simulink model "DYNctl_ver4_etud_obfusc"  (R2015a)
settings: Solver=ode45  StartTime=0.0  StopTime=tfin  FixedStep=0.001  RelTol=1e-09
values from neighbouring files (symbols this model uses):
  A_phi = [A13_13([1 4 11],1),A13_13([1 4 11],4),A13_13([1 4 11],11)]    [SM_4.m]
  A_theta = [A13_13([2 5 12],2),A13_13([2 5 12],5),A13_13([2 5 12],12)]    [SM_4.m]
  A_z = [A13_13([3 6 13],3),A13_13([3 6 13],6),A13_13([3 6 13],13)]    [SM_4.m]
  AxS = [A13_13([7 9],7),A13_13([7 9],9)]    [SM_4.m]
  AyS = [A13_13([8 10],8),A13_13([8 10],10)]    [SM_4.m]
  B_phi = [B13_3([1 4 11],1)]    [SM_4.m]
  B_theta = [B13_3([2 5 12],2)]    [SM_4.m]
  B_z = [B13_3([3 6 13],3)]    [SM_4.m]
  BxS = [0; acc]    [SM_4.m]
  ByS = [-acc; 0]    [SM_4.m]
  C3_3_iden = eye(3)    [SM_4.m]
  CxS = eye(2)    [SM_4.m]
  CyS = eye(2)    [SM_4.m]
  D_phi = [0;0;0]    [SM_4.m]
  D_theta = [0;0;0]    [SM_4.m]
  D_z = [0;0;0]    [SM_4.m]
  DxS = [0;0]    [SM_4.m]
  DyS = [0;0]    [SM_4.m]
  U_inv = 1/(YA*(-XB+XC)+YB*(XA-XC)+YC*(-XA+XB))*[-XB+XC, YC-YB, -YB*XC+YC*XB ... (first row only)    [SM_4.m]
  XA = r_ABC    (= 0.0952)    [SM-4.m]
  XB = -r_ABC*sind(30)    [SM-4.m]
  XC = 0    [SM-4.m]
  YA = 0    [SM-4.m]
  YB = r_ABC*cosd(30)    [SM-4.m]
  YC = -r_ABC*cosd(30)    [SM-4.m]
undefined symbols (not defined in the file or in its folder): ia_e, ib_e, ic_e, phi_e, TABC_trans, TDEF_trans, theta_e, va_e, vb_e, vc_e, vx_s_e, vy_s_e, vz_e, w_phi_e, w_theta_e, x_s_e, y_s_e, z_e
settings Model: CovSFcnEnable=off  Creator=delafontaine  LastModifiedBy=Julien
settings SolverCC: AlgebraicLoopSolver=LineSearch
settings DataIOCC: SignalLoggingSaveFormat=ModelDataLogs
settings DebuggingCC: UnderspecifiedInitializationDetection=Classic  MergeDetectMultiDrivingBlocksExec=none  MultiTaskDSMMsg=warning  MultiTaskCondExecSysMsg=none

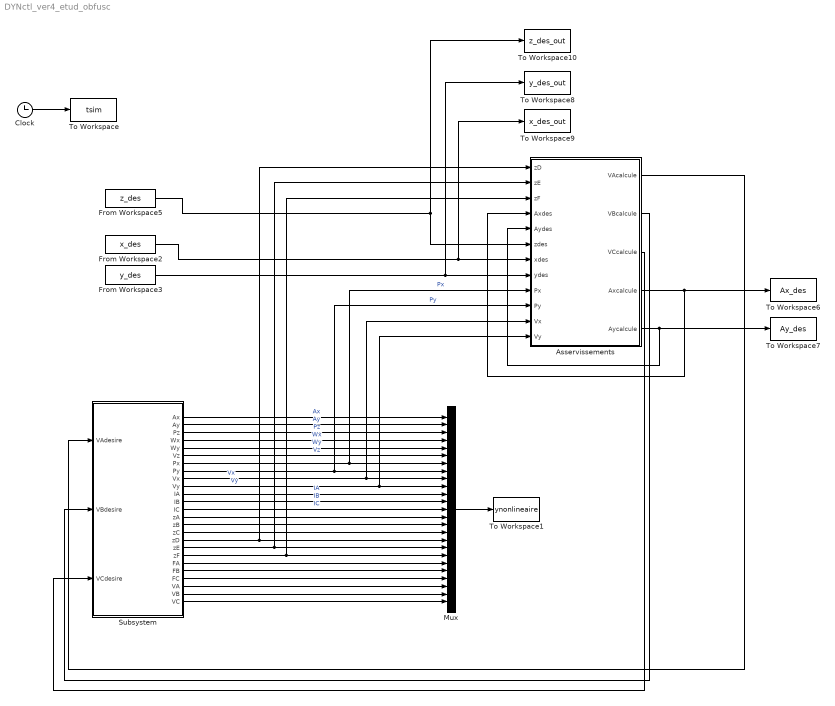
== system DYNctl_ver4_etud_obfusc ==
  Asservissements : Subsystem
      mask help: Simulink:masks:GenSFuncDesc_MD
      mask Help: eval('feval(''rtwprivate'',''rtwhelpview'',''rtw_sfcn_block'')');
  Clock : Clock
  From Workspace2 : FromWorkspace  VariableName=x_des  SampleTime=0  Interpolate=off  OutputAfterFinalValue=Holding final value
  From Workspace3 : FromWorkspace  VariableName=y_des  SampleTime=0  Interpolate=off  OutputAfterFinalValue=Holding final value
  From Workspace5 : FromWorkspace  VariableName=z_des  SampleTime=0  Interpolate=off  OutputAfterFinalValue=Holding final value
  Mux : Mux  Inputs=25
  Subsystem : Subsystem
  To Workspace : ToWorkspace  VariableName=tsim  SampleTime=-1
  To Workspace1 : ToWorkspace  VariableName=ynonlineaire  SampleTime=-1
  To Workspace10 : ToWorkspace  VariableName=z_des_out  SampleTime=-1
  To Workspace6 : ToWorkspace  VariableName=Ax_des  SampleTime=-1
  To Workspace7 : ToWorkspace  VariableName=Ay_des  SampleTime=-1
  To Workspace8 : ToWorkspace  VariableName=y_des_out  SampleTime=-1
  To Workspace9 : ToWorkspace  VariableName=x_des_out  SampleTime=-1
  wires:
  Mux/1 -> To Workspace1/1
  Clock/1 -> To Workspace/1
  From Workspace5/1 -> Asservissements/6(zdes), To Workspace10/1
  Subsystem/1(Ax) -> Mux/1  "Ax"
  Subsystem/2(Ay) -> Mux/2  "Ay"
  Subsystem/3(Pz) -> Mux/3  "Pz"
  Subsystem/4(Wx) -> Mux/4  "Wx"
  Subsystem/5(Wy) -> Mux/5  "Wy"
  Subsystem/6(Vz) -> Mux/6  "Vz"
  Subsystem/7(Px) -> Asservissements/9(Px), Mux/7  "Px"
  Subsystem/8(Py) -> Asservissements/10(Py), Mux/8  "Py"
  Subsystem/9(Vx) -> Asservissements/11(Vx), Mux/9  "Vx"
  Subsystem/10(Vy) -> Asservissements/12(Vy), Mux/10  "Vy"
  Subsystem/11(IA) -> Mux/11  "IA"
  Subsystem/12(IB) -> Mux/12  "IB"
  Subsystem/13(IC) -> Mux/13  "IC"
  From Workspace3/1 -> Asservissements/8(ydes), To Workspace8/1
  From Workspace2/1 -> Asservissements/7(xdes), To Workspace9/1
  Subsystem/20(FA) -> Mux/20
  Subsystem/21(FB) -> Mux/21
  Subsystem/22(FC) -> Mux/22
  Subsystem/23(VA) -> Mux/23
  Subsystem/24(VB) -> Mux/24
  Subsystem/25(VC) -> Mux/25
  Subsystem/17(zD) -> Asservissements/1(zD), Mux/17
  Subsystem/18(zE) -> Asservissements/2(zE), Mux/18
  Subsystem/19(zF) -> Asservissements/3(zF), Mux/19
  Subsystem/14(zA) -> Mux/14
  Subsystem/15(zB) -> Mux/15
  Subsystem/16(zC) -> Mux/16
  Asservissements/4(Axcalcule) -> Asservissements/4(Axdes), To Workspace6/1
  Asservissements/5(Aycalcule) -> Asservissements/5(Aydes), To Workspace7/1
  Asservissements/1(VAcalcule) -> Subsystem/1(VAdesire)
  Asservissements/2(VBcalcule) -> Subsystem/2(VBdesire)
  Asservissements/3(VCcalcule) -> Subsystem/3(VCdesire)

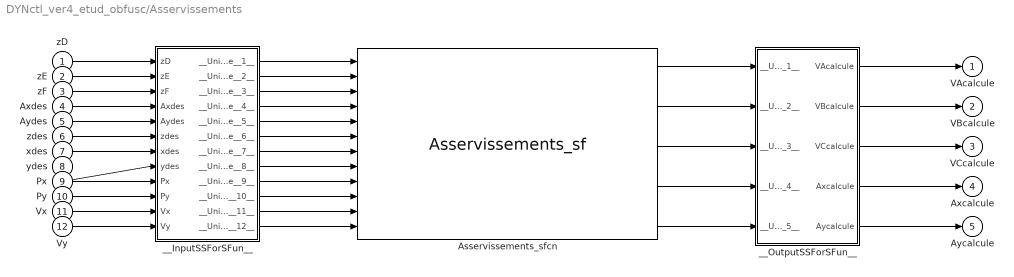
== system DYNctl_ver4_etud_obfusc/Asservissements ==
  zD : Inport
  zE : Inport  Port=2
  zF : Inport  Port=3
  Axdes : Inport  Port=4
  Aydes : Inport  Port=5
  zdes : Inport  Port=6
  xdes : Inport  Port=7
  ydes : Inport  Port=8
  Px : Inport  Port=9
  Py : Inport  Port=10
  Vx : Inport  Port=11
  Vy : Inport  Port=12
  Asservissements_sfcn : S-Function  FunctionName=Asservissements_sf  SFunctionModules=""  mask{rtw_sf_name=Asservissements_sf, showVar=off}
      mask prompts: rtw_sf_name "Simulink:masks:GenSFuncName_MP"; showVar "Simulink:masks:GenSFuncShowModuleList_MP"
      mask help: Simulink:masks:GenSFuncDesc_MD
      mask init:
      | displist = '';
      | if ~strcmp(get_param(gcb, 'FunctionName'), rtw_sf_name);
      |   set_param(gcb, 'FunctionName', rtw_sf_name);
      | end
      | % Check if we are generating code
      | rtw_mode = false;
      | if strcmpi(get_param(bdroot(gcb),'SimulationStatus'),'Initializing')
      | 	rtw_mode = strcmpi(get_param(bdroot(gcb),'BuildingRTWCode'),'on') && ...
      | 		~strcmpi(get_param(bdroot(gcb),'TargetStyle'),'SimulationTarget');
      | end
      | if showVar || rtw_mode
      | 	if exist('rtwsfunc') == 2 | exist('rtwsfunc') == 6
      | 		tmplist = rtwsfunc(rtw_sf_name,gcb);
      | 		tmplist = DAStudio.message('Simulink:masks:GenSFuncListOfModules_IC', tmplist);
      | 	elseif showVar
      | 		tmplist1 = DAStudio.message('Simulink:masks:GenSFuncListOfModules_IC', '');
      |         tmplist2 = DAStudio.message('Simulink:masks:GenSFuncNotLicensed_IC');
      |         tmplist = [tmplist1 tmplist2];
      |  	end
      | end
      | if showVar
      |   displist = tmplist;
      | end
      settings: CopyFcn=|
      | if ~strcmp(get_param(gcb,'Linkstatus'),'none') && ...
      | ~strcmp(get_param(gcb,'Linkstatus'),'implicit')
      |   set_param(gcb,'LinkStatus','none');
      | end
      mask Help: eval('feval(''rtwprivate'',''rtwhelpview'',''rtw_sfcn_block'')');
      mask Display:
      | port_label('input',1,'zD');
      | port_label('input',2,'zE');
      | port_label('input',3,'zF');
      | port_label('input',4,'Axdes');
      | port_label('input',5,'Aydes');
      | port_label('input',6,'zdes');
      | port_label('input',7,'xdes');
      | port_label('input',8,'ydes');
      | port_label('input',9,'Px');
      | port_label('input',10,'Py');
      | port_label('input',11,'Vx');
      | port_label('input',12,'Vy');
      | port_label('output',1,'VAcalcule');
      | port_label('output',2,'VBcalcule');
      | port_label('output',3,'VCcalcule');
      | port_label('output',4,'Axcalcule');
      | port_label('output',5,'Aycalcule');
  __InputSSForSFun__ : Subsystem
  __OutputSSForSFun__ : Subsystem
  VAcalcule : Outport
  VBcalcule : Outport  Port=2
  VCcalcule : Outport  Port=3
  Axcalcule : Outport  Port=4
  Aycalcule : Outport  Port=5
  wires:
  zD/1 -> __InputSSForSFun__/1(zD)
  zE/1 -> __InputSSForSFun__/2(zE)
  zF/1 -> __InputSSForSFun__/3(zF)
  Axdes/1 -> __InputSSForSFun__/4(Axdes)
  Aydes/1 -> __InputSSForSFun__/5(Aydes)
  zdes/1 -> __InputSSForSFun__/6(zdes)
  xdes/1 -> __InputSSForSFun__/7(xdes)
  ydes/1 -> __InputSSForSFun__/8(ydes)
  Px/1 -> __InputSSForSFun__/9(Px)
  Py/1 -> __InputSSForSFun__/10(Py)
  Vx/1 -> __InputSSForSFun__/11(Vx)
  Vy/1 -> __InputSSForSFun__/12(Vy)
  __InputSSForSFun__/1(__UniqueOutportName__1__) -> Asservissements_sfcn/1
  __InputSSForSFun__/2(__UniqueOutportName__2__) -> Asservissements_sfcn/2
  __InputSSForSFun__/3(__UniqueOutportName__3__) -> Asservissements_sfcn/3
  __InputSSForSFun__/4(__UniqueOutportName__4__) -> Asservissements_sfcn/4
  __InputSSForSFun__/5(__UniqueOutportName__5__) -> Asservissements_sfcn/5
  __InputSSForSFun__/6(__UniqueOutportName__6__) -> Asservissements_sfcn/6
  __InputSSForSFun__/7(__UniqueOutportName__7__) -> Asservissements_sfcn/7
  __InputSSForSFun__/8(__UniqueOutportName__8__) -> Asservissements_sfcn/8
  __InputSSForSFun__/9(__UniqueOutportName__9__) -> Asservissements_sfcn/9
  __InputSSForSFun__/10(__UniqueOutportName__10__) -> Asservissements_sfcn/10
  __InputSSForSFun__/11(__UniqueOutportName__11__) -> Asservissements_sfcn/11
  __InputSSForSFun__/12(__UniqueOutportName__12__) -> Asservissements_sfcn/12
  Asservissements_sfcn/1 -> __OutputSSForSFun__/1(__UniqueInportName__1__)
  Asservissements_sfcn/2 -> __OutputSSForSFun__/2(__UniqueInportName__2__)
  Asservissements_sfcn/3 -> __OutputSSForSFun__/3(__UniqueInportName__3__)
  Asservissements_sfcn/4 -> __OutputSSForSFun__/4(__UniqueInportName__4__)
  Asservissements_sfcn/5 -> __OutputSSForSFun__/5(__UniqueInportName__5__)
  __OutputSSForSFun__/1(VAcalcule) -> VAcalcule/1
  __OutputSSForSFun__/2(VBcalcule) -> VBcalcule/1
  __OutputSSForSFun__/3(VCcalcule) -> VCcalcule/1
  __OutputSSForSFun__/4(Axcalcule) -> Axcalcule/1
  __OutputSSForSFun__/5(Aycalcule) -> Aycalcule/1

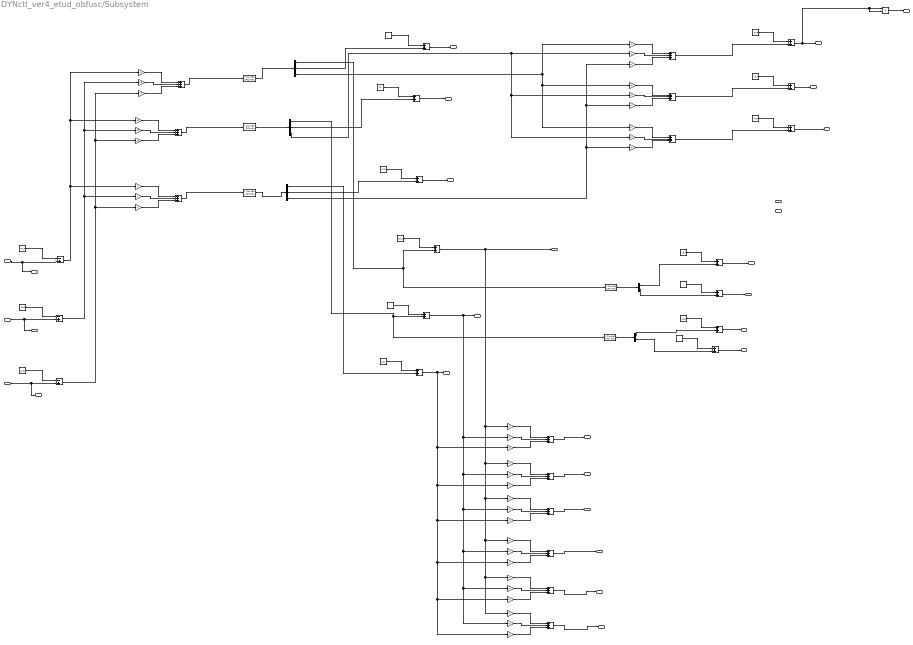
== system DYNctl_ver4_etud_obfusc/Subsystem ==
  note: za
  note: axe_x
  note: axe_y
  note: delta_phi
  note: delta_w_z
  note: delta_z_2
  note: delta_i_theta
  note: delta_theta_2
  note: delta_phi_2
  note: delta_phi
  note: delta_vb
  note: delta_z
  note: delta_theta
  note: bus_phi
  note: delat_df
  note: delta_vphi
  note: delta_vtheta
  note: delta_vz
  note: zb
  note: zc
  note: zd
  note: ze
  note: zf
  VAdesire : Inport
  VBdesire : Inport  Port=2
  VCdesire : Inport  Port=3
  Add : Sum  Inputs=-+
  Add1 : Sum  Inputs=-+
  Add{9..12,15..16,28..33} (12 alike) : Sum  Inputs=+++
  Add{13..14,17..27} (13 alike) : Sum
  Add2 : Sum  Inputs=-+
  Constant : Constant  Value=va_e
  Constant1 : Constant  Value=vb_e
  Constant10 : Constant  Value=z_e
  Constant11 : Constant  Value=vz_e
  Constant12 : Constant  Value=vy_s_e
  Constant13 : Constant  Value=y_s_e
  Constant14 : Constant  Value=x_s_e
  Constant15 : Constant  Value=vx_s_e
  Constant2 : Constant  Value=vc_e
  Constant3 : Constant  Value=ia_e
  Constant4 : Constant  Value=w_theta_e
  Constant5 : Constant  Value=w_phi_e
  Constant6 : Constant  Value=ib_e
  Constant7 : Constant  Value=ic_e
  Constant8 : Constant  Value=phi_e
  Constant9 : Constant  Value=theta_e
  Demux : Demux  Outputs=3
  Demux1 : Demux  Outputs=3
  Demux2 : Demux  Outputs=3
  Demux3 : Demux  Outputs=2
  Demux4 : Demux  Outputs=2
  Gain18 : Gain  Gain=YA
  Gain19 : Gain  Gain=YB
  Gain20 : Gain  Gain=YC
  Gain21 : Gain  Gain=-XA
  Gain22 : Gain  Gain=-XB
  Gain23 : Gain  Gain=-XC
  Gain24 : Gain
  Gain25 : Gain
  Gain26 : Gain
  Gain27 : Gain  Gain=U_inv(1,1)
  Gain28 : Gain  Gain=U_inv(1,2)
  Gain29 : Gain  Gain=U_inv(1,3)
  Gain30 : Gain  Gain=U_inv(2,1)
  Gain31 : Gain  Gain=U_inv(2,2)
  Gain32 : Gain  Gain=U_inv(2,3)
  Gain33 : Gain  Gain=U_inv(3,1)
  Gain34 : Gain  Gain=U_inv(3,2)
  Gain35 : Gain  Gain=U_inv(3,3)
  Gain36 : Gain  Gain=TABC_trans(1,1)
  Gain37 : Gain  Gain=TABC_trans(1,2)
  Gain38 : Gain  Gain=TABC_trans(1,3)
  Gain39 : Gain  Gain=TABC_trans(2,1)
  Gain40 : Gain  Gain=TABC_trans(2,2)
  Gain41 : Gain  Gain=TABC_trans(2,3)
  Gain42 : Gain  Gain=TABC_trans(3,1)
  Gain43 : Gain  Gain=TABC_trans(3,2)
  Gain44 : Gain  Gain=TABC_trans(3,3)
  Gain45 : Gain  Gain=TDEF_trans(1,1)
  Gain46 : Gain  Gain=TDEF_trans(1,2)
  Gain47 : Gain  Gain=TDEF_trans(1,3)
  Gain48 : Gain  Gain=TDEF_trans(2,1)
  Gain49 : Gain  Gain=TDEF_trans(2,2)
  Gain50 : Gain  Gain=TDEF_trans(2,3)
  Gain51 : Gain  Gain=TDEF_trans(3,1)
  Gain52 : Gain  Gain=TDEF_trans(3,2)
  Gain53 : Gain  Gain=TDEF_trans(3,3)
  Product : Product
  State-Space_phi1 : StateSpace  A=A_phi  B=B_phi  C=C3_3_iden  D=D_phi  X0=0
  State-Space_theta1 : StateSpace  A=A_theta  B=B_theta  C=C3_3_iden  D=D_theta  X0=0
  State-Space_xs : StateSpace  A=AxS  B=BxS  C=CxS  D=DxS  X0=0
  State-Space_ys : StateSpace  A=AyS  B=ByS  C=CyS  D=DyS  X0=0
  State-Space_z 1 : StateSpace  A=A_z  B=B_z  C=C3_3_iden  D=D_z  X0=0
  Ax : Outport
  Ay : Outport  Port=2
  Pz : Outport  Port=3
  Wx : Outport  Port=4
  Wy : Outport  Port=5
  Vz : Outport  Port=6
  Px : Outport  Port=7
  Py : Outport  Port=8
  Vx : Outport  Port=9
  Vy : Outport  Port=10
  IA : Outport  Port=11
  IB : Outport  Port=12
  IC : Outport  Port=13
  zA : Outport  Port=14
  zB : Outport  Port=15
  zC : Outport  Port=16
  zD : Outport  Port=17
  zE : Outport  Port=18
  zF : Outport  Port=19
  FA : Outport  Port=20
  FB : Outport  Port=21
  FC : Outport  Port=22
  VA : Outport  Port=23
  VB : Outport  Port=24
  VC : Outport  Port=25
  wires:
  Constant/1 -> Add/1
  VAdesire/1 -> VA/1, Add/2
  Constant2/1 -> Add2/1
  VCdesire/1 -> VC/1, Add2/2
  Constant1/1 -> Add1/1
  VBdesire/1 -> VB/1, Add1/2
  Demux2/1 -> Add23/2
  Gain18/1 -> Add9/1
  Gain19/1 -> Add9/2
  Gain20/1 -> Add9/3
  Add9/1 -> State-Space_phi1/1
  Add2/1 -> Gain23/1, Gain20/1, Gain26/1  "delta_vc"
  Gain21/1 -> Add10/1
  Gain22/1 -> Add10/2
  Gain23/1 -> Add10/3
  Add10/1 -> State-Space_theta1/1
  Add/1 -> Gain24/1, Gain21/1, Gain18/1  "delta_va"
  Add1/1 -> Gain25/1, Gain22/1, Gain19/1  "delta_vb"
  Gain24/1 -> Add11/1
  Gain25/1 -> Add11/2
  Gain26/1 -> Add11/3
  Add11/1 -> State-Space_z 1/1
  State-Space_phi1/1 -> Demux/1
  State-Space_theta1/1 -> Demux1/1  "delta_de"
  State-Space_z 1/1 -> Demux2/1
  Demux/2 -> Add14/2  "delta_w_phi"
  Demux1/2 -> Add13/2  "delta_w_theta"
  Demux2/2 -> Add20/2
  Constant4/1 -> Add13/1
  Constant5/1 -> Add14/1
  Constant11/1 -> Add20/1
  Add14/1 -> Wx/1
  Add13/1 -> Wy/1
  Add20/1 -> Vz/1
  Gain27/1 -> Add12/1
  Gain28/1 -> Add12/2
  Gain29/1 -> Add12/3
  Add12/1 -> Add17/2  "delta_ia"
  Gain30/1 -> Add15/1
  Gain31/1 -> Add15/2
  Gain32/1 -> Add15/3
  Add15/1 -> Add18/2  "delta_ib"
  Gain33/1 -> Add16/1
  Gain34/1 -> Add16/2
  Gain35/1 -> Add16/3
  Add16/1 -> Add19/2  "delta_ic"
  Demux/3 -> Gain27/1, Gain30/1, Gain33/1  "delta_i_phi"
  Demux1/3 -> Gain31/1, Gain34/1, Gain28/1  "delta_i_theta"
  Demux2/3 -> Gain35/1, Gain32/1, Gain29/1  "delta_i_z"
  Constant3/1 -> Add17/1
  Constant6/1 -> Add18/1
  Constant7/1 -> Add19/1
  Add18/1 -> IB/1
  Add19/1 -> IC/1
  Constant8/1 -> Add21/1
  Constant9/1 -> Add22/1
  Constant10/1 -> Add23/1
  Demux/1 -> Add21/2, State-Space_xs/1
  State-Space_xs/1 -> Demux3/1
  Demux1/1 -> State-Space_ys/1, Add22/2  "delta_theta"
  State-Space_ys/1 -> Demux4/1
  Demux3/1 -> Add25/2  "delta_ys"
  Demux3/2 -> Add24/2  "dela_vys"
  Demux4/1 -> Add26/2  "delta_xs"
  Demux4/2 -> Add27/2  "delta_vxs"
  Constant12/1 -> Add24/1
  Constant13/1 -> Add25/1
  Constant14/1 -> Add26/1
  Constant15/1 -> Add27/1
  Add25/1 -> Py/1
  Add24/1 -> Vy/1
  Add26/1 -> Px/1
  Add27/1 -> Vx/1
  Gain36/1 -> Add28/1
  Gain37/1 -> Add28/2
  Gain38/1 -> Add28/3
  Add28/1 -> zA/1
  Gain39/1 -> Add29/1
  Gain40/1 -> Add29/2
  Gain41/1 -> Add29/3
  Add29/1 -> zB/1
  Gain42/1 -> Add30/1
  Gain43/1 -> Add30/2
  Gain44/1 -> Add30/3
  Add30/1 -> zC/1
  Gain45/1 -> Add31/1
  Gain46/1 -> Add31/2
  Gain47/1 -> Add31/3
  Add31/1 -> zD/1
  Gain48/1 -> Add32/1
  Gain49/1 -> Add32/2
  Gain50/1 -> Add32/3
  Add21/1 -> Gain39/1, Gain42/1, Gain45/1, Gain48/1, Gain51/1, Gain36/1, Ax/1  "phi"
  Add32/1 -> zE/1
  Gain51/1 -> Add33/1
  Gain52/1 -> Add33/2
  Gain53/1 -> Add33/3
  Add22/1 -> Gain37/1, Gain52/1, Gain49/1, Gain46/1, Gain43/1, Gain40/1, Ay/1  "theta"
  Add23/1 -> Gain38/1, Gain41/1, Gain53/1, Gain50/1, Gain47/1, Gain44/1, Pz/1  "z"
  Add33/1 -> zF/1
  Add17/1 -> Product/2, Product/1, IA/1
  Product/1 -> FA/1

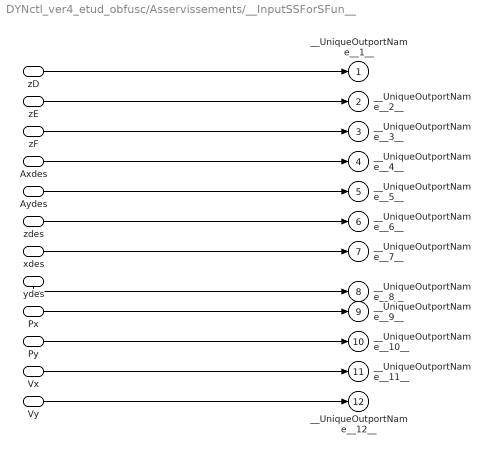
== system DYNctl_ver4_etud_obfusc/Asservissements/__InputSSForSFun__ ==
  zD : Inport
  zE : Inport  Port=2
  zF : Inport  Port=3
  Axdes : Inport  Port=4
  Aydes : Inport  Port=5
  zdes : Inport  Port=6
  xdes : Inport  Port=7
  ydes : Inport  Port=8
  Px : Inport  Port=9
  Py : Inport  Port=10
  Vx : Inport  Port=11
  Vy : Inport  Port=12
  __UniqueOutportName__1__ : Outport
  __UniqueOutportName__2__ : Outport  Port=2
  __UniqueOutportName__3__ : Outport  Port=3
  __UniqueOutportName__4__ : Outport  Port=4
  __UniqueOutportName__5__ : Outport  Port=5
  __UniqueOutportName__6__ : Outport  Port=6
  __UniqueOutportName__7__ : Outport  Port=7
  __UniqueOutportName__8__ : Outport  Port=8
  __UniqueOutportName__9__ : Outport  Port=9
  __UniqueOutportName__10__ : Outport  Port=10
  __UniqueOutportName__11__ : Outport  Port=11
  __UniqueOutportName__12__ : Outport  Port=12
  wires:
  zD/1 -> __UniqueOutportName__1__/1
  zE/1 -> __UniqueOutportName__2__/1
  zF/1 -> __UniqueOutportName__3__/1
  Axdes/1 -> __UniqueOutportName__4__/1
  Aydes/1 -> __UniqueOutportName__5__/1
  zdes/1 -> __UniqueOutportName__6__/1
  xdes/1 -> __UniqueOutportName__7__/1
  ydes/1 -> __UniqueOutportName__8__/1
  Px/1 -> __UniqueOutportName__9__/1
  Py/1 -> __UniqueOutportName__10__/1
  Vx/1 -> __UniqueOutportName__11__/1
  Vy/1 -> __UniqueOutportName__12__/1

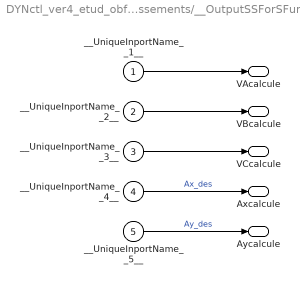
== system DYNctl_ver4_etud_obfusc/Asservissements/__OutputSSForSFun__ ==
  __UniqueInportName__1__ : Inport
  __UniqueInportName__2__ : Inport  Port=2
  __UniqueInportName__3__ : Inport  Port=3
  __UniqueInportName__4__ : Inport  Port=4
  __UniqueInportName__5__ : Inport  Port=5
  VAcalcule : Outport
  VBcalcule : Outport  Port=2
  VCcalcule : Outport  Port=3
  Axcalcule : Outport  Port=4
  Aycalcule : Outport  Port=5
  wires:
  __UniqueInportName__1__/1 -> VAcalcule/1
  __UniqueInportName__2__/1 -> VBcalcule/1
  __UniqueInportName__3__/1 -> VCcalcule/1
  __UniqueInportName__4__/1 -> Axcalcule/1  "Ax_des"
  __UniqueInportName__5__/1 -> Aycalcule/1  "Ay_des"
